simulink model "Tugas_no_2"  (R2022b)
settings: Solver=VariableStepAuto  StartTime=0.0  StopTime=10.0  RelTol=1e-3
settings Model: Creator=hp  LastModifiedBy=hp

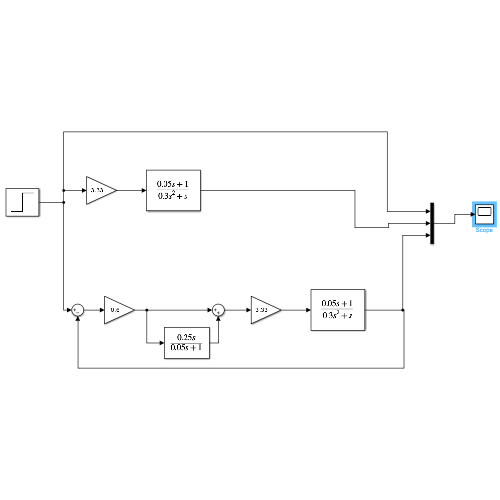
[thumbnail: Simulink's stored preview of the top-level diagram]
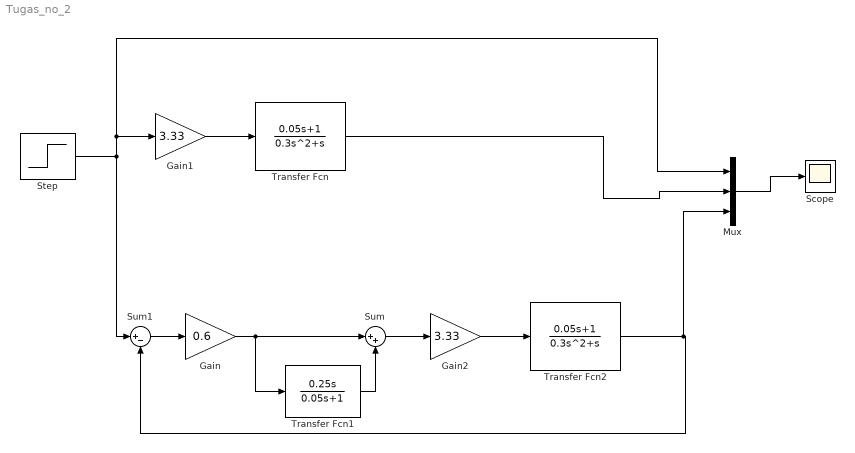
== system Tugas_no_2 ==
  Gain : Gain  Gain=0.6
  Gain1 : Gain  Gain=3.33
  Gain2 : Gain  Gain=3.33
  Mux : Mux  Inputs=3
  Scope : Scope
  Step : Step  SampleTime=0
  Sum : Sum  Inputs=|++
  Sum1 : Sum  Inputs=|+-
  Transfer Fcn : TransferFcn  Numerator=[0.05 1]  Denominator=[0.3 1 0]
  Transfer Fcn1 : TransferFcn  Numerator=[0.25 0]  Denominator=[0.05 1]
  Transfer Fcn2 : TransferFcn  Numerator=[0.05 1]  Denominator=[0.3 1 0]
  wires:
  Mux/1 -> Scope/1
  Gain/1 -> Transfer Fcn1/1, Sum/1
  Transfer Fcn1/1 -> Sum/2
  Sum1/1 -> Gain/1
  Gain1/1 -> Transfer Fcn/1
  Step/1 -> Mux/1, Gain1/1, Sum1/1
  Sum/1 -> Gain2/1
  Gain2/1 -> Transfer Fcn2/1
  Transfer Fcn2/1 -> Sum1/2, Mux/3
  Transfer Fcn/1 -> Mux/2
